simulink model "simple_subsystems"  (R2026a)
settings: Solver=ode1  StopTime=10  FixedStep=dt
model workspace (MAT data in the model file):
  D = Simulink.Parameter
  D.Value = 0
  D.Complexity = 'real'
  D.Dimensions = [1 1]
  D.DataType = 'auto'
  I = Simulink.Parameter
  I.Value = 1
  I.Complexity = 'real'
  I.Dimensions = [1 1]
  I.DataType = 'auto'
  P = Simulink.Parameter
  P.Value = 1
  P.Complexity = 'real'
  P.Dimensions = [1 1]
  P.DataType = 'auto'
  dt = Simulink.Parameter
  dt.Value = 0.001
  dt.Complexity = 'real'
  dt.Dimensions = [1 1]
  dt.Description = 'simulation time'
  dt.DataType = 'auto'
  dt.DocUnits = 'sec'
  setpoint = Simulink.Parameter
  setpoint.Value = 100
  setpoint.Complexity = 'real'
  setpoint.Dimensions = [1 1]
  setpoint.Description = 'setpoint for the experiment'
  setpoint.DataType = 'auto'
values from neighbouring files (symbols this model uses):
  D = 0    [simple_subsystems_parameters.m]
  dt = 0.001    [simple_subsystems_parameters.m]
  I = 1    [simple_subsystems_parameters.m]
  P = 1    [simple_subsystems_parameters.m]
  setpoint = 100    [simple_subsystems_parameters.m]
undefined symbols (not defined in the file or in its folder): DiscIntNeverNeededParam
libraries: slpidlib x1
settings Model: Creator=dcotterl  LastModifiedBy=dcotterl

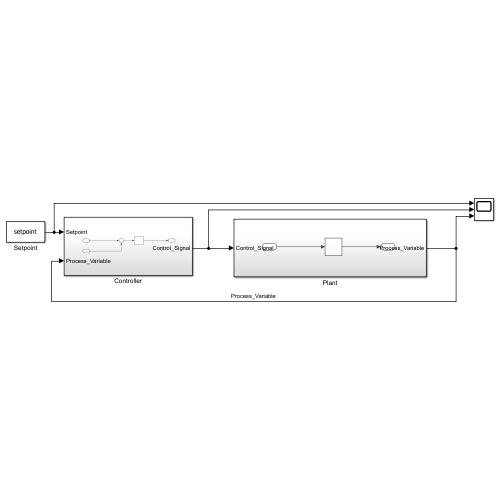
[thumbnail: Simulink's stored preview of the top-level diagram]
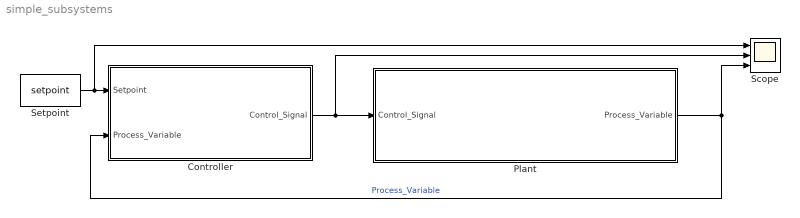
== system simple_subsystems ==
  Controller : Subsystem
  Plant : Subsystem
  Scope : Scope  NumInputPorts=3
      settings: ActiveDisplayYMinimum=-17.339312476895827  ActiveDisplayYMaximum=146.11468831406057
  Setpoint : Constant  Value=setpoint  VectorParams1D=off  OutDataTypeStr=double  SampleTime=dt
  wires:
  Plant/1(Process_Variable) -> Controller/2(Process_Variable), Scope/3  "Process_Variable"
  Setpoint/1 -> Scope/1, Controller/1(Setpoint)
  Controller/1(Control_Signal) -> Scope/2, Plant/1(Control_Signal)

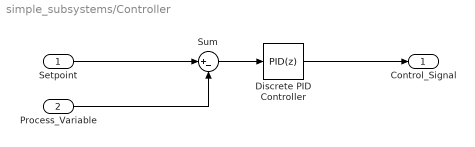
== system simple_subsystems/Controller ==
  Setpoint : Inport
  Process_Variable : Inport  Port=2
  Discrete PID Controller : slpidlib/PID Controller  Controller=PID  Form=Parallel  TimeDomain=Discrete-time  UseExternalTs=off  SampleTime=dt  IntegratorMethod=Forward Euler  FilterMethod=Forward Euler  ControllerParametersSource=internal  P=P  I=I  UseKiTs=off  D=D  UseExternalDerivativeSource=off  N=100  UseFilter=on  TunerSelectOption=Transfer Function Based (PID Tuner App)  InitialConditionSource=internal  InitialConditionForIntegrator=0  InitialConditionForFilter=0  DifferentiatorICPrevScaledInput=0  ExternalReset=none  TrackingMode=off  Kt=1  LimitOutput=off  SatLimitsSource=internal  UpperSaturationLimit=inf  LowerSaturationLimit=-inf  LinearizeAsGain=off  AntiWindupMode=none  Kb=1  LimitIntegrator=off  UpperIntegratorSaturationLimit=inf  LowerIntegratorSaturationLimit=-inf  PGainOutDataTypeStr=double  PProdOutDataTypeStr=double  POutMin=[]  POutMax=[]  IGainOutDataTypeStr=double  IProdOutDataTypeStr=double  IOutMin=[]  IOutMax=[]  DGainOutDataTypeStr=double  DProdOutDataTypeStr=double  DOutMin=[]  DOutMax=[]  NGainOutDataTypeStr=double  NProdOutDataTypeStr=double  NOutMin=[]  NOutMax=[]  SumOutDataTypeStr=double  SumOutMin=[]  SumOutMax=[]  SaturationOutMin=[]  SaturationOutMax=[]  PParamMin=[]  PParamMax=[]  IParamMin=[]  IParamMax=[]  DParamMin=[]  DParamMax=[]  NParamMin=[]  NParamMax=[]  KbParamMin=[]  KbParamMax=[]  KtParamMin=[]  KtParamMax=[]  KbOutMin=[]  KbOutMax=[]  KtOutMin=[]  KtOutMax=[]  IntegratorOutMin=[]  IntegratorOutMax=[]  FilterOutMin=[]  FilterOutMax=[]  SumI1OutMin=[]  SumI1OutMax=[]  SumI2OutMin=[]  SumI2OutMax=[]  SumI3OutMin=[]  SumI3OutMax=[]  SumI4OutMin=[]  SumI4OutMax=[]  SumDOutMin=[]  SumDOutMax=[]  DifferentiatorOutMin=[]  DifferentiatorOutMax=[]  FilterDiffOutCoefMin=[]  FilterDiffOutCoefMax=[]  ReciprocalOutMin=[]  ReciprocalOutMax=[]  SumDenOutMin=[]  SumDenOutMax=[]  SumNumOutMin=[]  SumNumOutMax=[]  DivideOutMin=[]  DivideOutMax=[]  UdiffTsProdOutMin=[]  UdiffTsProdOutMax=[]  NTsProdOutMin=[]  NTsProdOutMax=[]  UintegralTsProdOutMin=[]  UintegralTsProdOutMax=[]  UngainTsProdOutMin=[]  UngainTsProdOutMax=[]  ClampingZeroOutDataTypeStr=Inherit: Inherit via back propagation  ClampingZeroOutMin=[]  ClampingZeroOutMax=[]  FilterDenConstantOutDataTypeStr=Inherit: Inherit via back propagation  FilterDenConstantOutMin=[]  FilterDenConstantOutMax=[]  PCopyOutDataTypeStr=Inherit: Inherit via back propagation  PCopyOutMin=[]  PCopyOutMax=[]  NCopyOutDataTypeStr=Inherit: Inherit via back propagation  NCopyOutMin=[]  NCopyOutMax=[]  IntegratorContinuousStateAttributes=''  IntegratorStateMustResolveToSignalObject=off  IntegratorRTWStateStorageClass=Auto  FilterContinuousStateAttributes=''  FilterStateMustResolveToSignalObject=off  FilterRTWStateStorageClass=Auto  ParallelPVariant=InternalParameters  IdealPVariant=Disabled  IVariant=InternalParameters  DVariant=InternalParameters  IntegratorVariant=Discrete  SatVariant=Disabled  AWVariant=Passthrough  PCopyVariant=Disabled  TRVariant=Disabled  FdbkBlocksVariant=Forward  IdealPFdbkVariant=Disabled  SatFdbkVariant=Disabled  DerivativeFilterVariant=ForwardEulerFilter  NVariant=InternalParameters  NCopyVariant=Disabled  FilterICVariant=InternalICsFilter  IntegratorICVariant=InternalICs  ExternalResetVariant=Disabled  TRSumVariant=Passthrough  SumFdbkVariant=Disabled  SumVariant=Sum_PID  TsampFilterVariant=InternalTs  TsampNgainVariant=Passthrough  TsampIntegralVariant=Disabled_SignalSpec  ExternalSaturationOutDataTypeStr=Inherit: Same as second input  DerivativeSourceVariant=ErrorSignal  PreIntVariant=InternalPreInt
      settings: LibrarySourceBlock=simulink/Discrete/Discrete PID Controller
  Sum : Sum  Inputs=|+-  OutDataTypeStr=double  AccumDataTypeStr=double
  Control_Signal : Outport
  wires:
  Sum/1 -> Discrete PID Controller/1
  Setpoint/1 -> Sum/1
  Discrete PID Controller/1 -> Control_Signal/1
  Process_Variable/1 -> Sum/2

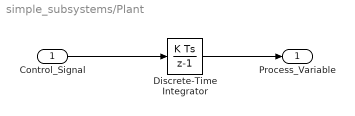
== system simple_subsystems/Plant ==
  Control_Signal : Inport
  Discrete-Time Integrator : DiscreteIntegrator  SampleTime=-1  ICPrevOutput=DiscIntNeverNeededParam  ICPrevScaledInput=DiscIntNeverNeededParam
  Process_Variable : Outport
  wires:
  Discrete-Time Integrator/1 -> Process_Variable/1
  Control_Signal/1 -> Discrete-Time Integrator/1
